simulink model "xmc_color_detection"  (R2020a)
settings: Solver=VariableStepAuto  StartTime=0.0  StopTime=inf  RelTol=1e-3
PostLoadFcn:
  | xmcHubUpdateInstalledDevice(gcs);
undefined symbols (not defined in the file or in its folder): gray, xc7vx485tffg1157
libraries: ModelComposer x12, color_detection_lib x8, xmcCopyrightNotice x1, dspvision x1
settings Model: Creator=ravalib  LastModifiedBy=viswanad
settings DataIOCC: ReturnWorkspaceOutputs=off
settings OptimizationCC: LifeSpan=inf
settings DebuggingCC: InheritedTsInSrcMsg=none  ArithmeticOperatorsInVariantConditions=warning
settings SFSimCC: SimUseLocalCustomCode=off  CustomCodeUndefinedFunction=UseInterfaceOnly
settings RTWCC: RTWUseLocalCustomCode=off
settings CodeAppCC: StateflowObjectComments=on

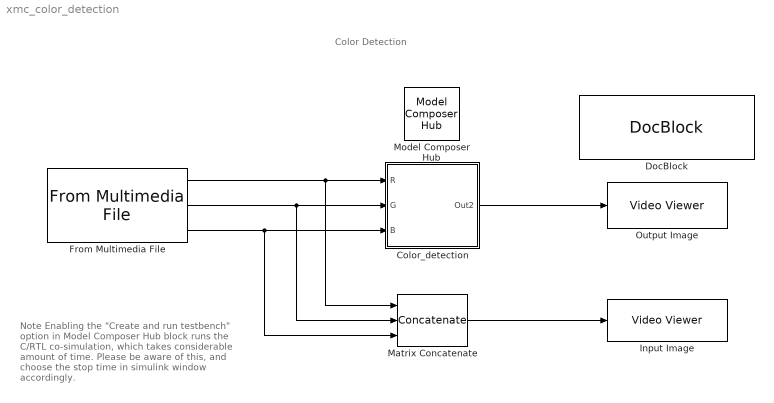
== system xmc_color_detection ==
  note: Color Detection
  note: Note
      |
      | Enabling the "Create and run testbench" option in Model Composer Hub block
      | runs the C/RTL co-simulation, which takes considerable amount of time.
      | Please be aware of this, and choose the stop time in simulink window accordingly.
  Color_detection : Subsystem
      mask Display: xmcDrawBlockIcon();
  DocBlock : xmcCopyrightNotice/DocBlock
      content=|
      | (c) Copyright 2017-2018 Xilinx, Inc. All rights reserved.
      |
      | This file contains confidential and proprietary information of Xilinx, Inc.
      | and is protected under U.S. and international copyright and other
      | intellectual property laws.
      |
      | DISCLAIMER
      | This disclaimer is not a license and does not grant any rights to the
      | materials distributed herewith. Except as otherwise provided in a valid
      | license issued to you by Xilinx, and to the maximum extent permitted by
      | applicable law: (1) THESE MATERIALS ARE MADE AVAILABLE "AS IS" AND WITH
      | ALL FAULTS, AND XILINX HEREBY DISCLAIMS ALL WARRANTIES AND CONDITIONS,
      | EXPRESS, IMPLIED, OR STATUTORY, INCLUDING BUT NOT LIMITED TO WARRANTIES
      | OF MERCHANTABILITY, NON-INFRINGEMENT, OR FITNESS FOR ANY PARTICULAR
      | PURPOSE; and (2) Xilinx shall not be liable (whether in contract or tort,
      | including negligence, or under any other theory of liability) for any
      | loss or damage of any kind or nature related to, arising under or in
      | connection with these materials, including for any direct, or any indirect,
      | special, incidental, or consequential loss or damage (including loss of
      | data, profits, goodwill, or any type of loss or damage suffered as a
      | result of any action brought by a third party) even if such damage or loss
      | was reasonably foreseeable or Xilinx had been advised of the possibility
      | of the same.
      |
      | CRITICAL APPLICATIONS
      | Xilinx products are not designed or intended to be fail-safe, or for use
      | in any application requiring fail-safe performance, such as life-support
      | or safety devices or systems, Class III medical devices, nuclear
      | facilities, applications related to the deployment of airbags, or
      | any other applications that could lead to death, personal injury, or
      | severe property or environmental damage (individually and collectively,
      | "Critical Applications"). Customer assumes the sole risk and liability
      | of any use of Xilinx products in Critical Applications, subject only to
      | applicable laws and regulations governing limitations on product liability.
      |
      | THIS COPYRIGHT NOTICE AND DISCLAIMER MUST BE RETAINED AS PART OF
      | THIS FILE AT ALL TIMES.
  From Multimedia File : dspvision/From Multimedia File  inputFilename=yellow_traffic_signs.avi  readRange=[1 Inf]  loop=on  numPlays=inf  outputStreams=Video only  videoDataType=uint8  audioDataType=int16  inheritSampleTime=off  userDefinedSampleTime=1/30  noAudioOutput=off  isIntensityVideo=off  fourcc=RGB  colorVideoFormat=Separate color signals  outputEOF=off  dataOrg=Column-major  audioFrameSize=1024  computeAudioFrameSize=off  outSamplingMode=Sample based
  Input Image : VideoViewer  colormapValue=gray(256)  FigPos=[425 718 1006 554]
  Matrix Concatenate : Concatenate  NumInputs=3  Mode=Multidimensional array  ConcatenateDimension=3
  Model Composer Hub : ModelComposer/Model Composer Hub  CodeGeneration=off  SubsystemName=Color_detection  TargetDirectory=./code  ExportType=IP Catalog  IpVendor=xilinx.com  IpLibrary=hls  IpVersion=1.0  IpHWLanguage=Verilog  AieCompilerOptions={}  CreateTestbench=off  TestbenchStackSize=10  RunAieSim=off  AieSimTimeout=50000  RunAieSimProfiling=off  LaunchVitisAnalyzer=off  PlotOutput=off  RunX86Sim=on  X86SimTimeout=10  GenHwImage=off  PlatformType=Not Specified  ProjDevice=xc7vx485tffg1157-1  ProjDevicePart=xc7vx485tffg1157-1  SamplePeriod=-1  ClockFrequency=200  DataPathParallelism=1
  Output Image : VideoViewer  colormapValue=gray(256)  FigPos=[33 747 919 556]
  wires:
  Matrix Concatenate/1 -> Input Image/1
  Color_detection/1(Out2) -> Output Image/1
  From Multimedia File/1 -> Matrix Concatenate/1, Color_detection/1(R)
  From Multimedia File/2 -> Matrix Concatenate/2, Color_detection/2(G)
  From Multimedia File/3 -> Matrix Concatenate/3, Color_detection/3(B)

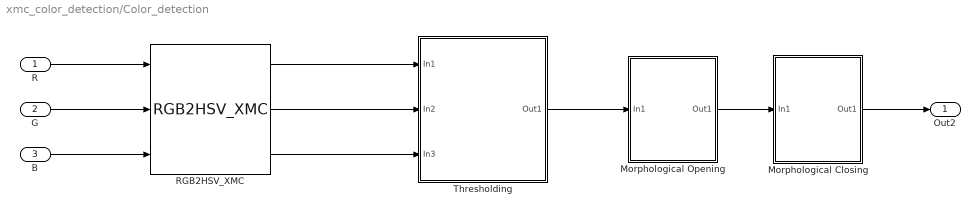
== system xmc_color_detection/Color_detection ==
  R : Inport
  G : Inport  Port=2
  B : Inport  Port=3
  Morphological Closing : Subsystem
      mask Display: xmcDrawBlockIcon();
  Morphological Opening : Subsystem
      mask Display: xmcDrawBlockIcon();
  RGB2HSV_XMC : color_detection_lib/RGB2HSV_XMC  LibraryFunction=RGB2HSV_XMC  IncludeFiles={'RGB2HSV_wrap.h'}  SourceFiles={}  IncludeDirectories={'./include'}  TemplateParams={'int ROWS'; 'int COLS'}  FunctionParamTypes={xmcDataType('void'); xmcDataType('uint8_t'); xmcDataType('uint8_t'); xmcDataType('uint8_t'); xmcDataType('uint8_t'); xmcDataType('uint8_t'); xmcDataType('uint8_t')}  FunctionParamPassbys={0.000000000000000000e+00; 0.000000000000000000e+00; 0.000000000000000000e+00; 0.000000000000000000e+00; 0.000000000000000000e+00; 0.000000000000000000e+00; 0.000000000000000000e+00}  FunctionParamDimensions={'1'; '[ROWS][COLS]'; '[ROWS][COLS]'; '[ROWS][COLS]'; '[ROWS][COLS]'; '[ROWS][COLS]'; '[ROWS][COLS]'}  FunctionParamNames={'return'; 'R'; 'G'; 'B'; 'H'; 'S'; 'V'}  FunctionParamDir={0.000000000000000000e+00; 1.000000000000000000e+00; 1.000000000000000000e+00; 1.000000000000000000e+00; 2.000000000000000000e+00; 2.000000000000000000e+00; 2.000000000000000000e+00}  FunctionParamSupportsStreaming={true; true; true; true; true; true; true}  BufferDepth={'0'}  FunctionParamValues={'0'; '0'; '0'; '0'; '0'; '0'; '0'}  ThroughputFactors={''}
  Thresholding : Subsystem  mask(Color Threshold){hue_low=20, hue_high=31, saturation_low=128, saturation_high=255, value_low=128, value_high=255}
      mask prompts: hue_low "Hue Low"; hue_high "Hue High"; saturation_low "Saturation Low"; saturation_high "Saturation High"; value_low "Value Low"; value_high "Value High"
      mask help: Compares the Hue, Saturation, and Value channels to the specificed threholds and renders a binary image.
      mask Help: Threshold Values should be between 0 and 255 inclusive. Use a phot editor tool to get the thresholds.
      mask DialogControl ParameterGroupVar Prompt: HSV Thresholds
      mask Display: xmcDrawBlockIcon();
  Out2 : Outport
  wires:
  RGB2HSV_XMC/2 -> Thresholding/2(In2)
  G/1 -> RGB2HSV_XMC/2
  Thresholding/1(Out1) -> Morphological Opening/1(In1)
  Morphological Opening/1(Out1) -> Morphological Closing/1(In1)
  Morphological Closing/1(Out1) -> Out2/1
  B/1 -> RGB2HSV_XMC/3
  R/1 -> RGB2HSV_XMC/1
  RGB2HSV_XMC/1 -> Thresholding/1(In1)
  RGB2HSV_XMC/3 -> Thresholding/3(In3)

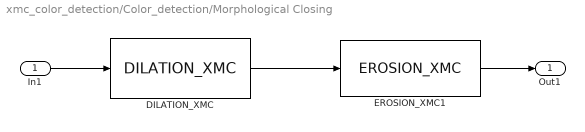
== system xmc_color_detection/Color_detection/Morphological Closing ==
  In1 : Inport
  DILATION_XMC : color_detection_lib/DILATION_XMC  LibraryFunction=DILATION_XMC  IncludeFiles={'DILATION_wrap.h'}  SourceFiles={}  IncludeDirectories={'./include'}  TemplateParams={'int ROWS'; 'int COLS'}  FunctionParamTypes={xmcDataType('void'); xmcDataType('uint8_t'); xmcDataType('uint8_t'); xmcDataType('unsigned char')}  FunctionParamPassbys={0.000000000000000000e+00; 0.000000000000000000e+00; 0.000000000000000000e+00; 0.000000000000000000e+00}  FunctionParamDimensions={'1'; '[ROWS][COLS]'; '[ROWS][COLS]'; '[9]'}  FunctionParamNames={'return'; 'src'; 'dst'; 'kernel'}  FunctionParamDir={0.000000000000000000e+00; 1.000000000000000000e+00; 2.000000000000000000e+00; 3.000000000000000000e+00}  FunctionParamSupportsStreaming={true; true; true; true}  BufferDepth={'0'}  FunctionParamValues={'0'; '0'; '0'; '0'}  ThroughputFactors={''}  kernel=[1 1 1 1 1 1 1 1 1]
  EROSION_XMC1 : color_detection_lib/EROSION_XMC  LibraryFunction=EROSION_XMC  IncludeFiles={'EROSION_wrap.h'}  SourceFiles={}  IncludeDirectories={'./include'}  TemplateParams={'int ROWS'; 'int COLS'}  FunctionParamTypes={xmcDataType('void'); xmcDataType('uint8_t'); xmcDataType('uint8_t'); xmcDataType('unsigned char')}  FunctionParamPassbys={0.000000000000000000e+00; 0.000000000000000000e+00; 0.000000000000000000e+00; 0.000000000000000000e+00}  FunctionParamDimensions={'1'; '[ROWS][COLS]'; '[ROWS][COLS]'; '[9]'}  FunctionParamNames={'return'; 'src'; 'dst'; 'kernel'}  FunctionParamDir={0.000000000000000000e+00; 1.000000000000000000e+00; 2.000000000000000000e+00; 3.000000000000000000e+00}  FunctionParamSupportsStreaming={true; true; true; true}  BufferDepth={'0'}  FunctionParamValues={'0'; '0'; '0'; '0'}  ThroughputFactors={''}  kernel=[1 1 1 1 1 1 1 1 1]
  Out1 : Outport
  wires:
  DILATION_XMC/1 -> EROSION_XMC1/1
  In1/1 -> DILATION_XMC/1
  EROSION_XMC1/1 -> Out1/1

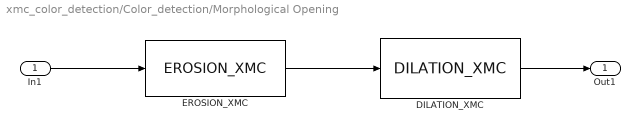
== system xmc_color_detection/Color_detection/Morphological Opening ==
  In1 : Inport
  DILATION_XMC : color_detection_lib/DILATION_XMC  LibraryFunction=DILATION_XMC  IncludeFiles={'DILATION_wrap.h'}  SourceFiles={}  IncludeDirectories={'./include'}  TemplateParams={'int ROWS'; 'int COLS'}  FunctionParamTypes={xmcDataType('void'); xmcDataType('uint8_t'); xmcDataType('uint8_t'); xmcDataType('unsigned char')}  FunctionParamPassbys={0.000000000000000000e+00; 0.000000000000000000e+00; 0.000000000000000000e+00; 0.000000000000000000e+00}  FunctionParamDimensions={'1'; '[ROWS][COLS]'; '[ROWS][COLS]'; '[9]'}  FunctionParamNames={'return'; 'src'; 'dst'; 'kernel'}  FunctionParamDir={0.000000000000000000e+00; 1.000000000000000000e+00; 2.000000000000000000e+00; 3.000000000000000000e+00}  FunctionParamSupportsStreaming={true; true; true; true}  BufferDepth={'0'}  FunctionParamValues={'0'; '0'; '0'; '0'}  ThroughputFactors={''}  kernel=[1 1 1 1 1 1 1 1 1]
  EROSION_XMC : color_detection_lib/EROSION_XMC  LibraryFunction=EROSION_XMC  IncludeFiles={'EROSION_wrap.h'}  SourceFiles={}  IncludeDirectories={'./include'}  TemplateParams={'int ROWS'; 'int COLS'}  FunctionParamTypes={xmcDataType('void'); xmcDataType('uint8_t'); xmcDataType('uint8_t'); xmcDataType('unsigned char')}  FunctionParamPassbys={0.000000000000000000e+00; 0.000000000000000000e+00; 0.000000000000000000e+00; 0.000000000000000000e+00}  FunctionParamDimensions={'1'; '[ROWS][COLS]'; '[ROWS][COLS]'; '[9]'}  FunctionParamNames={'return'; 'src'; 'dst'; 'kernel'}  FunctionParamDir={0.000000000000000000e+00; 1.000000000000000000e+00; 2.000000000000000000e+00; 3.000000000000000000e+00}  FunctionParamSupportsStreaming={true; true; true; true}  BufferDepth={'0'}  FunctionParamValues={'0'; '0'; '0'; '0'}  ThroughputFactors={''}  kernel=[1 1 1 1 1 1 1 1 1]
  Out1 : Outport
  wires:
  EROSION_XMC/1 -> DILATION_XMC/1
  In1/1 -> EROSION_XMC/1
  DILATION_XMC/1 -> Out1/1

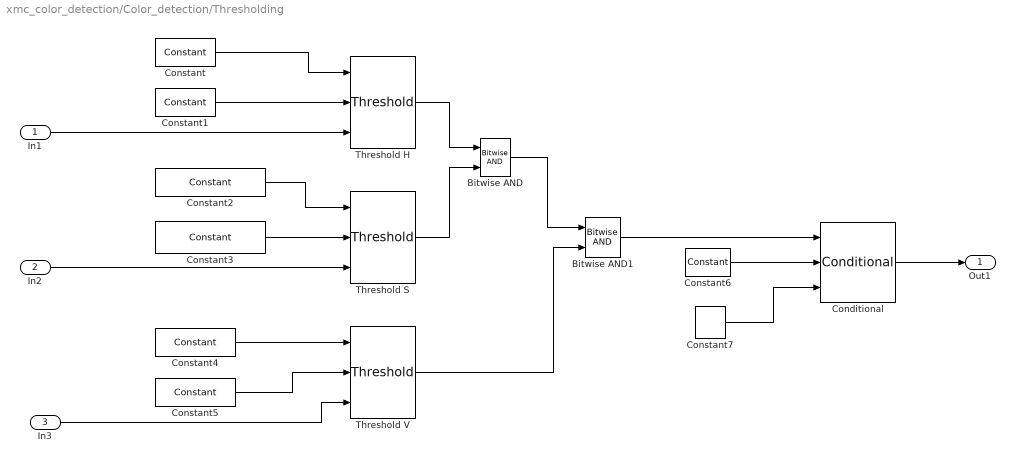
== system xmc_color_detection/Color_detection/Thresholding ==
  In1 : Inport
  In2 : Inport  Port=2
  In3 : Inport  Port=3
  Bitwise AND : ModelComposer/Bitwise AND
  Bitwise AND1 : ModelComposer/Bitwise AND
  Conditional : ModelComposer/Conditional  Condition=C ~= 0  Threshold=0.00
  Constant : ModelComposer/Constant  Value=hue_low  VectorParams1D=off  SampleTime=-1  OutDataType=uint8  TypeExp=''  Signedness=Signed  WordLength=16  FractionalLength=0  RoundingMode=Truncation to minus infinity  OverflowMode=Wrap around
  Constant1 : ModelComposer/Constant  Value=hue_high  VectorParams1D=off  SampleTime=-1  OutDataType=uint8  TypeExp=''  Signedness=Signed  WordLength=16  FractionalLength=0  RoundingMode=Truncation to minus infinity  OverflowMode=Wrap around
  Constant2 : ModelComposer/Constant  Value=saturation_low  VectorParams1D=off  SampleTime=-1  OutDataType=uint8  TypeExp=''  Signedness=Signed  WordLength=16  FractionalLength=0  RoundingMode=Truncation to minus infinity  OverflowMode=Wrap around
  Constant3 : ModelComposer/Constant  Value=saturation_high  VectorParams1D=off  SampleTime=-1  OutDataType=uint8  TypeExp=''  Signedness=Signed  WordLength=16  FractionalLength=0  RoundingMode=Truncation to minus infinity  OverflowMode=Wrap around
  Constant4 : ModelComposer/Constant  Value=value_low  VectorParams1D=off  SampleTime=-1  OutDataType=uint8  TypeExp=''  Signedness=Signed  WordLength=16  FractionalLength=0  RoundingMode=Truncation to minus infinity  OverflowMode=Wrap around
  Constant5 : ModelComposer/Constant  Value=value_high  VectorParams1D=off  SampleTime=-1  OutDataType=uint8  TypeExp=''  Signedness=Signed  WordLength=16  FractionalLength=0  RoundingMode=Truncation to minus infinity  OverflowMode=Wrap around
  Constant6 : ModelComposer/Constant  Value=1  VectorParams1D=off  SampleTime=-1  OutDataType=uint8  TypeExp=''  Signedness=Signed  WordLength=16  FractionalLength=0  RoundingMode=Truncation to minus infinity  OverflowMode=Wrap around
  Constant7 : ModelComposer/Constant  Value=0  VectorParams1D=off  SampleTime=-1  OutDataType=uint8  TypeExp=''  Signedness=Signed  WordLength=16  FractionalLength=0  RoundingMode=Truncation to minus infinity  OverflowMode=Wrap around
  Threshold H : color_detection_lib/Threshold  SystemSampleTime=-1  Latency=0  AutoFrameSizeCalculation=off
  Threshold S : color_detection_lib/Threshold  SystemSampleTime=-1  Latency=0  AutoFrameSizeCalculation=off
  Threshold V : color_detection_lib/Threshold  SystemSampleTime=-1  Latency=0  AutoFrameSizeCalculation=off
  Out1 : Outport
  wires:
  Conditional/1 -> Out1/1
  Bitwise AND1/1 -> Conditional/1
  Constant6/1 -> Conditional/2
  Constant7/1 -> Conditional/3
  Threshold S/1 -> Bitwise AND/2
  Constant5/1 -> Threshold V/2
  In2/1 -> Threshold S/3
  Constant2/1 -> Threshold S/1
  Threshold V/1 -> Bitwise AND1/2
  In3/1 -> Threshold V/3
  Threshold H/1 -> Bitwise AND/1
  Constant3/1 -> Threshold S/2
  In1/1 -> Threshold H/3
  Constant4/1 -> Threshold V/1
  Bitwise AND/1 -> Bitwise AND1/1
  Constant1/1 -> Threshold H/2
  Constant/1 -> Threshold H/1
